simulink model "chap9_6"  (Simulink 3.00)
settings: Solver=ode45  StartTime=0  StopTime=5  RelTol=1e-3
values from neighbouring files (symbols this model uses):
  bc = 30.0    (= 30)    [Chap9_5i.m]    (also in chap9_6i.m = 3)
  bl = 8.0    (= 8)    [chap9_6i.m]
  bm = 0.010    (= 0.01)    [chap9_6i.m]
  Ce = 0.001    [Chap9_5i.m]    (also in chap9_3.m = 1.2; chap9_4plant.m = 1.2; chap9_6i.m)
  Fc = 15    [CHAP9_3F.M]    (also in Chap9_5i.m = 100; chap9_1eq.m = 0.28; chap9_2s.m = 0.28; chap9_4plant.m)
  Jl = 0.15    [chap9_6i.m]
  Jm = 0.005    [chap9_6i.m]
  kd = 6    [Chap9_5i.m]    (also in chap9_6i.m; chap9_7i.m)
  kdd = 1.5    [Chap9_5i.m]    (also in chap9_6i.m = 5)
  ki = 0.001    [Chap9_5i.m]    (also in chap9_6i.m)
  kii = 0.1    [Chap9_5i.m]    (also in chap9_6i.m = 1)
  kl = 5.0    (= 5)    [chap9_6i.m]
  km = 1.0    (= 1)    [Chap9_5i.m]    (also in chap9_6i.m = 10)
  kpp = 150    [Chap9_5i.m]    (also in chap9_6i.m = 8)
  ku = 11    [Chap9_5i.m]    (also in chap9_6i.m)
  kv = 2.0    (= 2)    [CHAP9_3F.M]    (also in Chap9_5i.m; chap9_4plant.m; chap9_6i.m; chap9_7i.m)
  L = 0.001    [Chap9_5i.m]    (also in chap9_6i.m)
  R = 1    [Chap9_5i.m]    (also in chap9_3.m = 7.77; chap9_4plant.m = 7.77; chap9_6i.m)
undefined symbols (not defined in the file or in its folder): sgn
libraries: simulink_extras x1

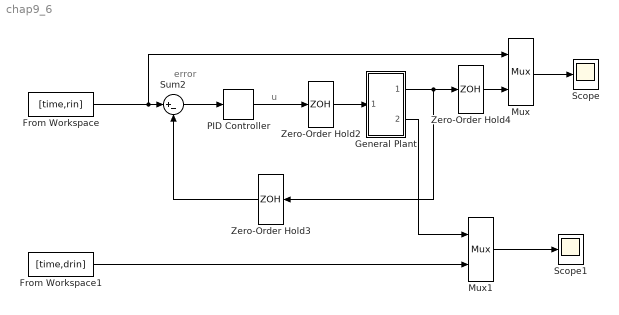
== system chap9_6 ==
  note: u
  note: error
  From Workspace : FromWorkspace  VariableName=[time,rin]  SampleTime=0.001  HoldFinalValue=off
  From Workspace1 : FromWorkspace  VariableName=[time,drin]  SampleTime=0.001  HoldFinalValue=off
  General Plant : Subsystem
  Mux : Mux  Inputs=2
      settings: DisplayOption=none
  Mux1 : Mux  Inputs=2
      settings: DisplayOption=none
  PID Controller : simulink_extras/Additional Linear/PID Controller  P=kpp  I=kii  D=kdd
  Scope : Scope
      settings: TimeRange=auto  YMin=-0.5  YMax=0.5  SaveToWorkspace=off  SaveName=ScopeData  MaxRows=50000
  Scope1 : Scope
      settings: TimeRange=auto  YMin=-1.75  YMax=1.75  SaveToWorkspace=off  SaveName=ScopeData  MaxRows=500000
  Sum2 : Sum  Inputs=|+-  SaturateOnIntegerOverflow=on
  Zero-Order Hold2 : ZeroOrderHold  SampleTime=0.001
  Zero-Order Hold3 : ZeroOrderHold  Orientation=left  SampleTime=0.001
  Zero-Order Hold4 : ZeroOrderHold  SampleTime=0.001
  wires:
  Mux/1 -> Scope/1
  Zero-Order Hold4/1 -> Mux/2
  Zero-Order Hold2/1 -> General Plant/1(In1)
  Mux1/1 -> Scope1/1
  General Plant/1(Out1) -> Zero-Order Hold3/1, Zero-Order Hold4/1
  General Plant/2(Out2) -> Mux1/1
  Sum2/1 -> PID Controller/1
  Zero-Order Hold3/1 -> Sum2/2
  From Workspace/1 -> Sum2/1, Mux/1
  PID Controller/1 -> Zero-Order Hold2/1
  From Workspace1/1 -> Mux1/2

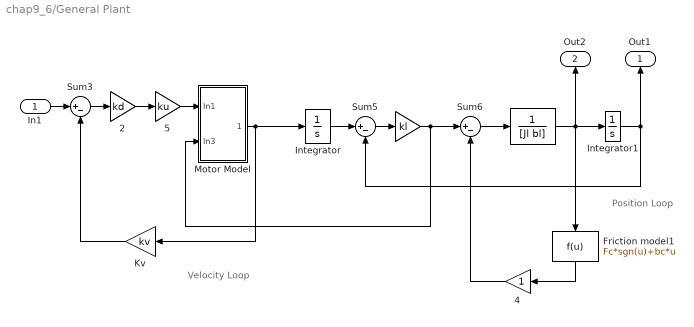
== system chap9_6/General Plant ==
  note: Velocity Loop
  note: Position Loop
  In1 : Inport  Port=1  PortWidth=-1  SampleTime=-1  DataType=auto
      settings: SignalType=auto
  " " : Gain  Gain=kl  SaturateOnIntegerOverflow=on
  "    " : TransferFcn  Numerator=[1]  Denominator=[Jl bl]
  " 2" : Gain  Gain=kd  SaturateOnIntegerOverflow=on
  " 4" : Gain  Orientation=left  Gain=1  SaturateOnIntegerOverflow=on
  " 5" : Gain  Gain=ku  SaturateOnIntegerOverflow=on
  Friction model1 : Fcn  Orientation=down  Expr=Fc*sgn(u)+bc*u
  Integrator : Integrator  ExternalReset=none  InitialConditionSource=internal  InitialCondition=0  LimitOutput=off  UpperSaturationLimit=inf  LowerSaturationLimit=-inf  ShowSaturationPort=off  ShowStatePort=off  AbsoluteTolerance=auto
  Integrator1 : Integrator  ExternalReset=none  InitialConditionSource=internal  InitialCondition=0  LimitOutput=off  UpperSaturationLimit=inf  LowerSaturationLimit=-inf  ShowSaturationPort=off  ShowStatePort=off  AbsoluteTolerance=auto
  Kv : Gain  Orientation=left  Gain=kv  SaturateOnIntegerOverflow=on
  Motor Model : Subsystem
  Sum3 : Sum  Inputs=|+-  SaturateOnIntegerOverflow=on
  Sum5 : Sum  Inputs=|+-  SaturateOnIntegerOverflow=on
  Sum6 : Sum  Inputs=|+-  SaturateOnIntegerOverflow=on
  Out1 : Outport  Orientation=up  Port=1
  Out2 : Outport  Orientation=up  Port=2
  wires:
  Kv/1 -> Sum3/2
  Motor Model/1(Out1) -> Integrator/1, Kv/1
  In1/1 -> Sum3/1
  Sum3/1 -> " 2"/1
  " 2"/1 -> " 5"/1
  " 5"/1 -> Motor Model/1(In1)
  Sum5/1 -> " "/1
  Integrator/1 -> Sum5/1
  Integrator1/1 -> Sum5/2, Out1/1
  Sum6/1 -> "    "/1
  " "/1 -> Sum6/1, Motor Model/2(In3)
  "    "/1 -> Friction model1/1, Integrator1/1, Out2/1
  Friction model1/1 -> " 4"/1
  " 4"/1 -> Sum6/2

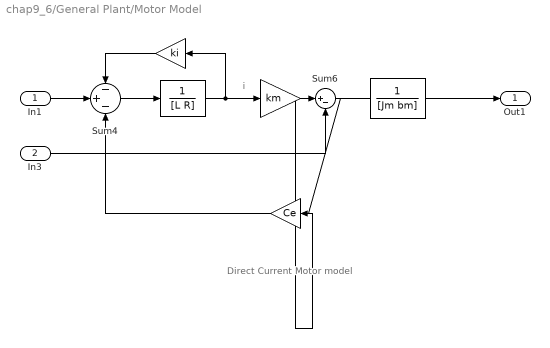
== system chap9_6/General Plant/Motor Model ==
  note: i
  note: Direct Current Motor model
  In1 : Inport  Port=1  PortWidth=-1  SampleTime=-1  DataType=auto
      settings: SignalType=auto
  In3 : Inport  Port=2  PortWidth=-1  SampleTime=-1  DataType=auto
      settings: SignalType=auto
  "    " : Gain  Orientation=left  Gain=Ce  SaturateOnIntegerOverflow=on
  "      " : Gain  Orientation=left  Gain=ki  SaturateOnIntegerOverflow=on
  "  " : Gain  Gain=km  SaturateOnIntegerOverflow=on
  "   " : TransferFcn  Numerator=[1]  Denominator=[L R]
  "    " : TransferFcn  Numerator=[1]  Denominator=[Jm bm]
  Sum4 : Sum  Inputs=-+-  SaturateOnIntegerOverflow=off
  Sum6 : Sum  Inputs=|+-  SaturateOnIntegerOverflow=on
  Out1 : Outport  Port=1
  wires:
  "    "/1 -> "    "/1, Out1/1
  Sum4/1 -> "   "/1
  "   "/1 -> "      "/1, "  "/1
  "      "/1 -> Sum4/1
  In1/1 -> Sum4/2
  "  "/1 -> Sum6/1
  In3/1 -> Sum6/2
  "    "/1 -> Sum4/3
  Sum6/1 -> "    "/1
